simulink model "rover_ros_io"  (R2024b)
settings: Solver=FixedStepAuto  StartTime=0.0  StopTime=inf  FixedStep=0.1  RelTol=1e-3
StartFcn:
  | simulink_teleop_start();
StopFcn:
  | simulink_teleop_stop();
undefined symbols (not defined in the file): angular, linear, simulink_teleop_ang, simulink_teleop_lin
libraries: ros2lib x4
settings Model: Creator=dinuk  LastModifiedBy=dinuk

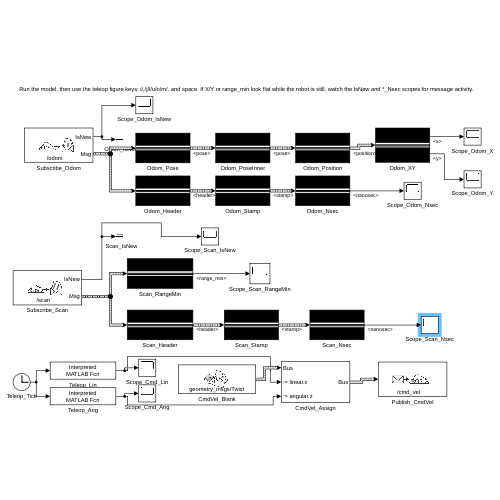
[thumbnail: Simulink's stored preview of the top-level diagram]
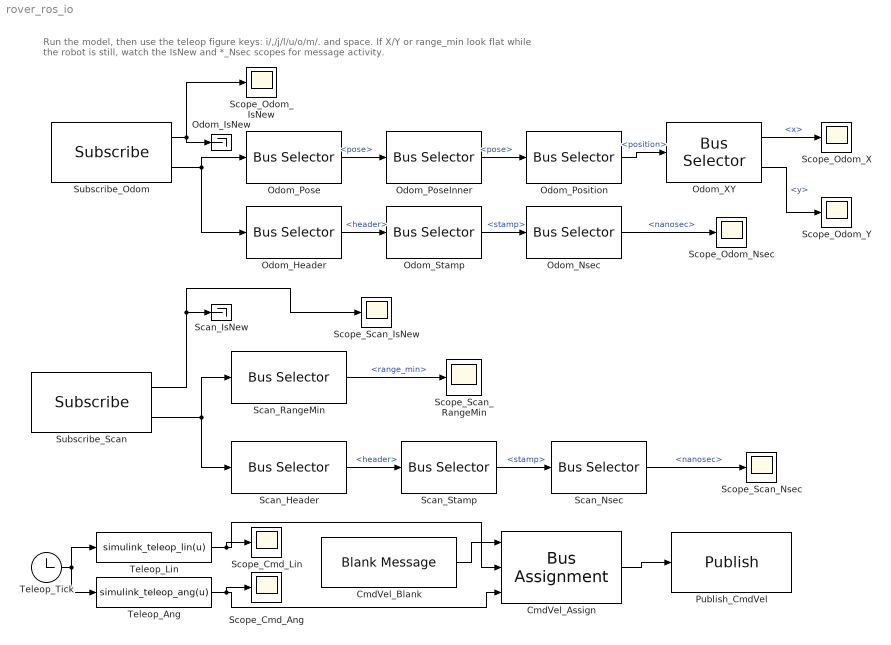
== system rover_ros_io ==
  note: Run the model, then use the teleop figure keys: i/,/j/l/u/o/m/. and space. If X/Y or range_min look flat while the robot is still, watch the IsNew and *_Nsec scopes for message activity.
  CmdVel_Assign : BusAssignment  AssignedSignals=linear.x,angular.z
  CmdVel_Blank : ros2lib/Blank Message  messageClass=Message  entityType=geometry_msgs/Twist  messageType=geometry_msgs/Twist  SampleTime=0.1
      link override Constant: OutDataTypeStr=Bus: SL_Bus_geometry_msgs_Twist
  Odom_Header : BusSelector  OutputSignals=header
  Odom_IsNew : Terminator
  Odom_Nsec : BusSelector  OutputSignals=nanosec
  Odom_Pose : BusSelector  OutputSignals=pose
  Odom_PoseInner : BusSelector  OutputSignals=pose
  Odom_Position : BusSelector  OutputSignals=position
  Odom_Stamp : BusSelector  OutputSignals=stamp
  Odom_XY : BusSelector  OutputSignals=x,y
  Publish_CmdVel : ros2lib/Publish  topicSource=Specify your own  topic=/cmd_vel  messageType=geometry_msgs/Twist  QOSHistory=Keep last  QOSDepth=10  QOSReliability=Reliable  QOSDurability=Volatile  QOSDeadline=Inf  QOSLifespan=Inf  QOSLiveliness=Automatic  QOSLeaseDuration=Inf  QOSAvoidROSNamespaceConventions=off
      link override SignalSpecification: OutDataTypeStr=Bus: SL_Bus_geometry_msgs_Twist
      link override SinkBlock: ROSTopic=/cmd_vel  ROSMessageType=geometry_msgs/Twist  SLBusName=SL_Bus_geometry_msgs_Twist  ModelName=rover_ros_io  BlockId=Pub_rover_ros_io_31
  Scan_Header : BusSelector  OutputSignals=header
  Scan_IsNew : Terminator
  Scan_Nsec : BusSelector  OutputSignals=nanosec
  Scan_RangeMin : BusSelector  OutputSignals=range_min
  Scan_Stamp : BusSelector  OutputSignals=stamp
  Scope_Cmd_Ang : Scope
  Scope_Cmd_Lin : Scope
  Scope_Odom_IsNew : Scope
  Scope_Odom_Nsec : Scope
  Scope_Odom_X : Scope
  Scope_Odom_Y : Scope
  Scope_Scan_IsNew : Scope
  Scope_Scan_Nsec : Scope
  Scope_Scan_RangeMin : Scope
  Subscribe_Odom : ros2lib/Subscribe  topicSource=Specify your own  topic=/odom  messageType=nav_msgs/Odometry  sampleTime=0.1  QOSHistory=Keep last  QOSDepth=10  QOSReliability=Reliable  QOSDurability=Volatile  QOSDeadline=Inf  QOSLifespan=Inf  QOSLiveliness=Automatic  QOSLeaseDuration=Inf  QOSAvoidROSNamespaceConventions=off
      link override Constant: OutDataTypeStr=Bus: SL_Bus_nav_msgs_Odometry
      link override SourceBlock: ROSTopic=/odom  ROSMessageType=nav_msgs/Odometry  SLBusName=SL_Bus_nav_msgs_Odometry  ModelName=rover_ros_io  BlockId=Sub_rover_ros_io_2
  Subscribe_Scan : ros2lib/Subscribe  topicSource=Specify your own  topic=/scan  messageType=sensor_msgs/LaserScan  sampleTime=0.1  QOSHistory=Keep last  QOSDepth=10  QOSReliability=Best effort  QOSDurability=Volatile  QOSDeadline=Inf  QOSLifespan=Inf  QOSLiveliness=Automatic  QOSLeaseDuration=Inf  QOSAvoidROSNamespaceConventions=off
      link override Constant: OutDataTypeStr=Bus: SL_Bus_sensor_msgs_LaserScan
      link override SourceBlock: ROSTopic=/scan  ROSMessageType=sensor_msgs/LaserScan  SLBusName=SL_Bus_sensor_msgs_LaserScan  ModelName=rover_ros_io  BlockId=Sub_rover_ros_io_15
  Teleop_Ang : MATLABFcn  MATLABFcn=simulink_teleop_ang(u)
  Teleop_Lin : MATLABFcn  MATLABFcn=simulink_teleop_lin(u)
  Teleop_Tick : Clock
  wires:
  Subscribe_Odom/1 -> Scope_Odom_IsNew/1, Odom_IsNew/1
  Subscribe_Odom/2 -> Odom_Pose/1, Odom_Header/1
  Odom_Header/1 -> Odom_Stamp/1  "<header>"
  Odom_Stamp/1 -> Odom_Nsec/1  "<stamp>"
  Odom_Nsec/1 -> Scope_Odom_Nsec/1  "<nanosec>"
  Odom_Pose/1 -> Odom_PoseInner/1  "<pose>"
  Odom_PoseInner/1 -> Odom_Position/1  "<pose>"
  Odom_Position/1 -> Odom_XY/1  "<position>"
  Odom_XY/1 -> Scope_Odom_X/1  "<x>"
  Odom_XY/2 -> Scope_Odom_Y/1  "<y>"
  Subscribe_Scan/1 -> Scope_Scan_IsNew/1, Scan_IsNew/1
  Subscribe_Scan/2 -> Scan_RangeMin/1, Scan_Header/1
  Scan_Header/1 -> Scan_Stamp/1  "<header>"
  Scan_Stamp/1 -> Scan_Nsec/1  "<stamp>"
  Scan_Nsec/1 -> Scope_Scan_Nsec/1  "<nanosec>"
  Scan_RangeMin/1 -> Scope_Scan_RangeMin/1  "<range_min>"
  Teleop_Tick/1 -> Teleop_Lin/1, Teleop_Ang/1
  Teleop_Lin/1 -> Scope_Cmd_Lin/1, CmdVel_Assign/2
  Teleop_Ang/1 -> Scope_Cmd_Ang/1, CmdVel_Assign/3
  CmdVel_Blank/1 -> CmdVel_Assign/1
  CmdVel_Assign/1 -> Publish_CmdVel/1
